simulink model "Copy_of_SIMSCAPE_SIM_PROTOTYPE"  (R2024b)
settings: Solver=ode15s  StartTime=0.0  StopTime=T_sim  MaxStep=1e-6  RelTol=1e-6
InitFcn:
  | run param_file.m
  | % param = struct();
  | %
  | % % Pressure Rails
  | % param.P_T = 101325;
  | % param.P_H = 7e6;
  | % param.P_M = 3.5e6;
  | % param.P_L = param.P_T;
  | %
  | % % Linear Actuator Chamber
  | % param.V1_0 = 250e-6;
  | % param.Acap = pi*(2.54)^2*1e-4;
  | %
  | % % Intermediary volumes
  | % param.V3_0 = 10e-6;
  | % param.V4_0 = 10e-6;
  | %
  | % % Fluid
  | % param.beta = 1.8e9;
  | % param.air = 0;
  | % param.rho = 870;
  | %
  | % % Valve
  | % param.max_Avt = 4.9160e-06;
  | % param.Cd = 0.6;
  | % param.stroke = 5e-3;
  | %
  | % % Valve Dynamics
  | % param.wn = 50*2*pi;
  | % param.zeta = 1;
  | %
  | % % Hydraulic Pump/Motor
  | % param.J_hyd = 3000e-7;
  | % param.D = 0.8e-6;    % In cc/rev
  | % param.pump_mech_eff = 100*(1/100);
  | % param.pump_vol_eff = 100*(1/100);
  | %
  | % % Electric Motor/Generator
  | % param.J_elec = 3060e-7;
  | % param.Kt = 109e-3;
  | % param.Kv = (88*pi)/30; % In rads^-1/Volt
  | % param.elec_eff = 100*(1/100);
  | % param.max_mech_power = 90;
  | %
  | % % Initial speed
  | % param.start_final_velocity = 100;
values from neighbouring files (symbols this model uses):
  param = struct()    [Copy_of_param_file.m]    (also in param_file.m; param_file_loss_vs_freq.m; param_file_original.m; param_file_turbine.m)
libraries: fl_lib x42, nesl_utility x28, SimscapeFluids_lib x4, ee_lib x3, eeDcCurrentController x1, eePwmGenerator x1
(part 2 of 2)

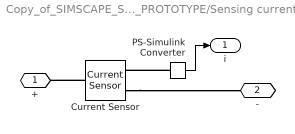
== system Copy_of_SIMSCAPE_SIM_PROTOTYPE/Sensing current ==
  Current Sensor : fl_lib/Electrical/Electrical Sensors/Current Sensor
  PS-Simulink Converter : nesl_utility/PS-Simulink Converter  PhysicalDomain=network_engine_domain  SubClassName=ps_output  LeftPortType=input  RightPortType=output  PseudoPeriodic=off  Frequencies=[]  VectorFormat=1-D array  Unit=1  AffineConversion=off
  + : PMIOPort  Side=Left
  - : PMIOPort  Port=2  Side=Right
  i : Outport
  wires:
  PS-Simulink Converter/1 -> i/1
  connections:
  PS-Simulink Converter/LConn1 -- Current Sensor/RConn1
  Current Sensor/RConn2 -- -/RConn1
  Current Sensor/LConn1 -- +/RConn1

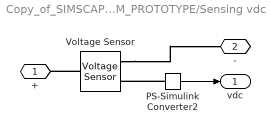
== system Copy_of_SIMSCAPE_SIM_PROTOTYPE/Sensing vdc ==
  PS-Simulink Converter2 : nesl_utility/PS-Simulink Converter  PhysicalDomain=network_engine_domain  SubClassName=ps_output  LeftPortType=input  RightPortType=output  PseudoPeriodic=off  Frequencies=[]  VectorFormat=1-D array  Unit=V  AffineConversion=off
  Voltage Sensor : fl_lib/Electrical/Electrical Sensors/Voltage Sensor
  + : PMIOPort  Side=Left
  - : PMIOPort  Port=2  Side=Right
  vdc : Outport
  wires:
  PS-Simulink Converter2/1 -> vdc/1
  connections:
  Voltage Sensor/LConn1 -- +/RConn1
  PS-Simulink Converter2/LConn1 -- Voltage Sensor/RConn1
  Voltage Sensor/RConn2 -- -/RConn1

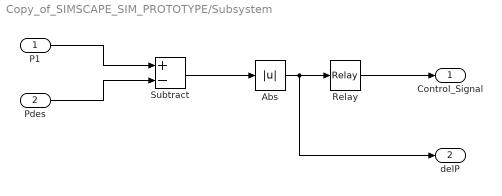
== system Copy_of_SIMSCAPE_SIM_PROTOTYPE/Subsystem ==
  P1 : Inport
  Pdes : Inport  Port=2
  Abs : Abs  SaturateOnIntegerOverflow=off
  Relay : Relay  OnSwitchValue=6e5  OffSwitchValue=1e4  OnOutputValue=0  OffOutputValue=1
  Subtract : Sum  Inputs=+-
  Control_Signal : Outport
  delP : Outport  Port=2
  wires:
  P1/1 -> Subtract/1
  Pdes/1 -> Subtract/2
  Subtract/1 -> Abs/1
  Abs/1 -> delP/1, Relay/1
  Relay/1 -> Control_Signal/1

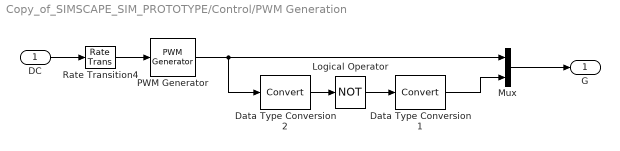
== system Copy_of_SIMSCAPE_SIM_PROTOTYPE/Control/PWM Generation ==
  DC : Inport
  Data Type Conversion1 : DataTypeConversion  SaturateOnIntegerOverflow=off  RndMeth=Floor
  Data Type Conversion2 : DataTypeConversion  SaturateOnIntegerOverflow=off  RndMeth=Floor
  Logical Operator : Logic  Operator=NOT  AllPortsSameDT=off  OutDataTypeStr=boolean
  Mux : Mux  Inputs=2
  PWM Generator : eePwmGenerator/PWM Generator  CarrCount=Up  Tper=1/1e7  Tdelay=0  Ts=1e-8
  Rate Transition4 : RateTransition  OutPortSampleTimeOpt=Inherit  OutPortSampleTime=Ts
  G : Outport  VectorParamsAs1DForOutWhenUnconnected=off
  wires:
  Data Type Conversion2/1 -> Logical Operator/1
  DC/1 -> Rate Transition4/1
  PWM Generator/1 -> Mux/1, Data Type Conversion2/1
  Logical Operator/1 -> Data Type Conversion1/1
  Data Type Conversion1/1 -> Mux/2
  Mux/1 -> G/1
  Rate Transition4/1 -> PWM Generator/1

== matlab function Copy_of_SIMSCAPE_SIM_PROTOTYPE/Electric Torque Controller1 ==
  data: Control_Signal input; Kp input; omega input; T_elec output; start_final_velocity input; T_elec_max input
function T_elec  = fcn(Control_Signal, Kp, omega, start_final_velocity, T_elec_max)

if Control_Signal == 1 

    if omega < start_final_velocity
        omega_error = omega -start_final_velocity;
        
        T_elec = - (Kp*omega_error);

    else
        T_elec = -T_elec_max;
    end

else

    if omega >= 124.99
        omega_error = omega -125;
        T_elec = -(Kp*omega_error);

    else
        T_elec = T_elec_max;
    end

end

== matlab function Copy_of_SIMSCAPE_SIM_PROTOTYPE/MATLAB Function ==
  data: Power_loss_2 output; P_A_big input; P1 input; P_P_small input; P_T_small input; S_small input; Q_A_big input; Qout input
function Power_loss_2 = fcn(P_A_big, P1, P_P_small, P_T_small, S_small, Q_A_big, Qout)

Power_loss_2 = (S_small>2.5e-3)*((P_A_big-P_P_small)*Q_A_big + (P_T_small-P1)*Qout) ...
              +(S_small<-2.5e-3)*((P_A_big-P_T_small)*Q_A_big + (P_P_small-P1)*Qout)...
              +(S_small>=-2.5e-3 && S_small<=2.5e-3)*((P_A_big-P_P_small)*Q_A_big + (P_T_small-P1)*Qout + (P_A_big-P_T_small)*Q_A_big + (P_P_small-P1)*Qout);

== matlab function Copy_of_SIMSCAPE_SIM_PROTOTYPE/MATLAB Function2 ==
  data: Pdes input; S_big output; S_small output; param parameter; Control_signal input
function [S_big, S_small] = fcn(Pdes, param, Control_signal)

if Pdes == param.P_H && Control_signal == 0
    S_big = param.stroke;
    S_small = param.stroke;
elseif Pdes == param.P_M && Control_signal == 0
    S_big = -param.stroke;
    S_small = -param.stroke;
elseif Pdes == param.P_H && Control_signal > 0
    S_big = param.stroke;
    S_small = 0;
elseif Pdes == param.P_M && Control_signal > 0
    S_big = -param.stroke;
    S_small = 0;
else
    S_big = 0;
    S_small = 0;
end

== matlab function Copy_of_SIMSCAPE_SIM_PROTOTYPE/MATLAB Function4 ==
  data: P_H_rail input; P_M_rail input; Q_P_big input; Q_T_big input; Power_out_1 output; Power_out_2 output
function [Power_out_1, Power_out_2] = fcn(P_H_rail, P_M_rail, Q_P_big, Q_T_big)

Power_out_1 = (Q_P_big)*(P_H_rail);

Power_out_2 = (Q_T_big)*(P_M_rail);

== matlab function Copy_of_SIMSCAPE_SIM_PROTOTYPE/MATLAB Function1 ==
  data: P1 input; Qout input; Power_out output; param parameter
function Power_out = fcn(P1, Qout, param)

gamma = 1.4; % Adiabatic process
Pt = param.P_T;

Pg = P1-Pt;   % Gauge pressure
r = P1/Pt;    % Pressure ratio
e = exp(Pg/param.beta);
rv = (1/e+param.air*r^(-1/gamma))/(1+param.air);      %Volume ratio

El=param.beta*(e-(1+Pg/param.beta))+Pt*(e-1);           %Energy in liquid
Eg=P1/(gamma-1).*(1-r.^(1/gamma-1));          %Energy in gas
E=(El./e+param.air*Eg.*r.^(-1/gamma))./(1./e+param.air*r.^(-1/gamma));    %Energy in mixture
W = E-(1./rv-1)*Pt;  %Compressibility (volumetric) energy density

Power_out = (Qout)*(W+Pg);
